simulink model "Bitwise"  (R2021a)
settings: Solver=VariableStepAuto  StartTime=0.0  StopTime=10.0  RelTol=1e-3
settings Model: Creator=elkny  LastModifiedBy=elkny

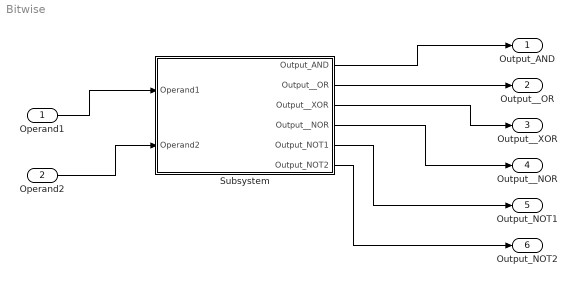
== system Bitwise ==
  Operand1 : Inport
  Operand2 : Inport  Port=2
  Subsystem : Subsystem
  Output_AND : Outport
  Output__OR : Outport  Port=2
  Output__XOR : Outport  Port=3
  Output__NOR : Outport  Port=4
  Output_NOT1 : Outport  Port=5
  Output_NOT2 : Outport  Port=6
  wires:
  Operand1/1 -> Subsystem/1(Operand1)
  Operand2/1 -> Subsystem/2(Operand2)
  Subsystem/1(Output_AND) -> Output_AND/1
  Subsystem/2(Output__OR) -> Output__OR/1
  Subsystem/3(Output__XOR) -> Output__XOR/1
  Subsystem/4(Output__NOR) -> Output__NOR/1
  Subsystem/5(Output_NOT1) -> Output_NOT1/1
  Subsystem/6(Output_NOT2) -> Output_NOT2/1

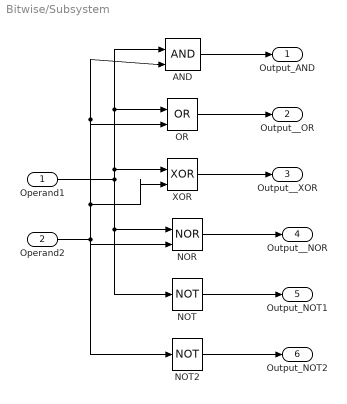
== system Bitwise/Subsystem ==
  Operand1 : Inport
  Operand2 : Inport  Port=2
  AND : Logic  IconShape=distinctive  AllPortsSameDT=off  OutDataTypeStr=boolean
  NOR : Logic  Operator=NOR  IconShape=distinctive  AllPortsSameDT=off  OutDataTypeStr=boolean
  NOT : Logic  Operator=NOT  IconShape=distinctive  AllPortsSameDT=off  OutDataTypeStr=boolean
  NOT2 : Logic  Operator=NOT  IconShape=distinctive  AllPortsSameDT=off  OutDataTypeStr=boolean
  OR : Logic  Operator=OR  IconShape=distinctive  AllPortsSameDT=off  OutDataTypeStr=boolean
  XOR : Logic  Operator=XOR  IconShape=distinctive  AllPortsSameDT=off  OutDataTypeStr=boolean
  Output_AND : Outport
  Output__OR : Outport  Port=2
  Output__XOR : Outport  Port=3
  Output__NOR : Outport  Port=4
  Output_NOT1 : Outport  Port=5
  Output_NOT2 : Outport  Port=6
  wires:
  Operand1/1 -> NOT/1, NOR/1, XOR/1, OR/1, AND/1
  OR/1 -> Output__OR/1
  Operand2/1 -> NOT2/1, NOR/2, XOR/2, OR/2, AND/2
  AND/1 -> Output_AND/1
  NOT2/1 -> Output_NOT2/1
  XOR/1 -> Output__XOR/1
  NOT/1 -> Output_NOT1/1
  NOR/1 -> Output__NOR/1
